simulink model "Sliding_mode"  (R2020b)
settings: Solver=VariableStepAuto  StartTime=0.0  StopTime=50  RelTol=1e-3
settings Model: Creator=zhiyao  LastModifiedBy=zhiyao

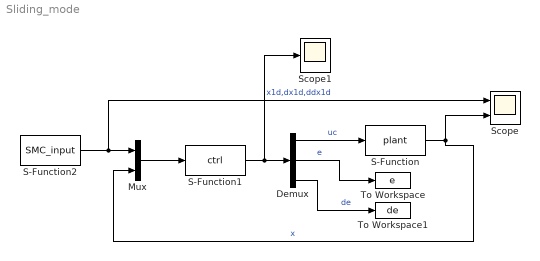
== system Sliding_mode ==
  Demux : Demux  Outputs=3
  Mux : Mux  Inputs=2
  S-Function : S-Function  FunctionName=plant  Parameters=pa  SFunctionDeploymentMode=off  EnableBusSupport=off
  S-Function1 : S-Function  FunctionName=ctrl  Parameters=pa  SFunctionDeploymentMode=off  EnableBusSupport=off
  S-Function2 : S-Function  FunctionName=SMC_input  Parameters=pa  SFunctionDeploymentMode=off  EnableBusSupport=off
  Scope : Scope  NumInputPorts=2
  Scope1 : Scope
  To Workspace : ToWorkspace  VariableName=e  SampleTime=-1
  To Workspace1 : ToWorkspace  VariableName=de  SampleTime=-1
  wires:
  S-Function1/1 -> Demux/1, Scope1/1
  S-Function2/1 -> Scope/1, Mux/1  "x1d,dx1d,ddx1d"
  S-Function/1 -> Mux/2, Scope/2  "x"
  Mux/1 -> S-Function1/1
  Demux/1 -> S-Function/1  "uc"
  Demux/2 -> To Workspace/1  "e"
  Demux/3 -> To Workspace1/1  "de"
